simulink model "ECS_FOS"  (Simulink 8.2)
settings: Solver=ode45  StartTime=0.0  StopTime=18000  RelTol=1e-3
InitFcn:
  | load('loss_coeff_mixing_junction.mat')
  | load('SampleOutput.mat')
  | load('HydProp.mat')
  | load('HydraulicLoad.mat')
  | load('initavload.mat')
  | load('SampleFuelBurn.mat')
values from neighbouring files (symbols this model uses):
  FuelBurn = [0 0 0 0 0 0 0 0 0 0 0 0 ... (18249 elements, 1x18249)]    [Benchmark_data1.mat]
  fueltankdata =     [Benchmark_data1.mat]
undefined symbols (not defined in the file or in its folder): AirProp, F1, F2, HUGHES_TREITLER, magnitude, PN_70147, PumpProp
libraries: PowerFlowLib x46, simulink x4
(part 2 of 5)

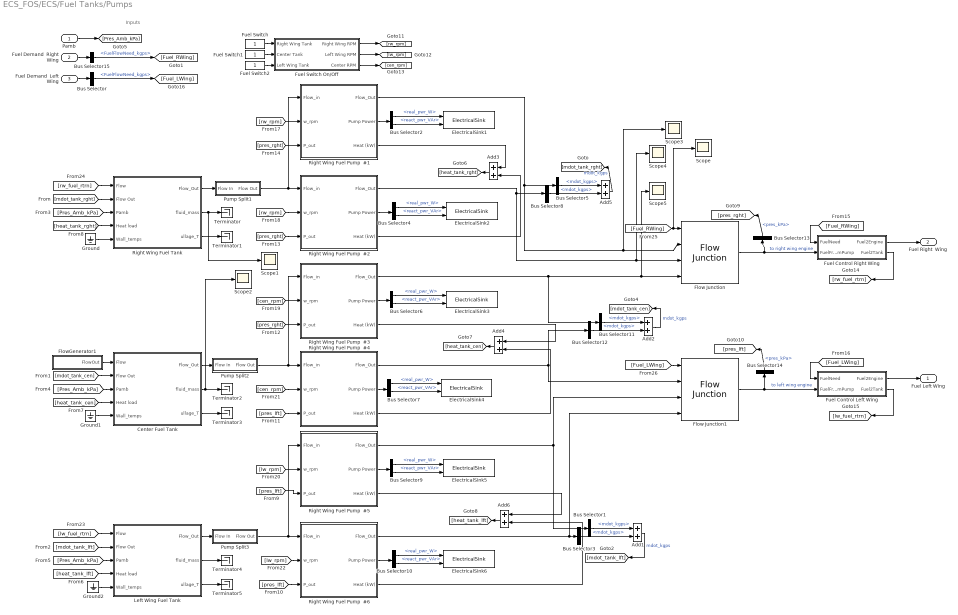
== system ECS_FOS/ECS/Fuel Tanks/Pumps ==
  note: Inputs
  Pamb : Inport
  Fuel Demand  Right Wing : Inport  Port=2
  Fuel Demand  Left Wing : Inport  Port=3
  Add{1..6} (6 alike) : Sum
  Bus Selector : BusSelector  OutputSignals=Fuel.FuelFlowNeed_kgps
  Bus Selector{1,3,5,8,11..12} (6 alike) : BusSelector  OutputSignals=mdot_kgps
  Bus Selector{2,4,6..7,9..10} (6 alike) : BusSelector  OutputSignals=real_pwr_W,react_pwr_VAr
  Bus Selector13 : BusSelector  OutputSignals=pres_kPa
  Bus Selector14 : BusSelector  OutputSignals=pres_kPa
  Bus Selector15 : BusSelector  OutputSignals=Fuel.FuelFlowNeed_kgps
  Center Fuel Tank : Subsystem  AncestorBlock=PowerFlowLib/Energy & Power Systems/Thermal/Fuel/Fuel Tank  mask(Fuel Tank){fileslct=off, filename=fueltank_area.m, filedir=C:\Users\mwillms4\Documents\My Box Files\Graduate\Research\PowerFlow Development\PowerFlow Fall 2013\SupportFunctions\fueltank_area.m, tank_loc=Center Tank, areaprompt2=off, max_vol=3.2, m_init=2500, fld_Tint=0, ull_Tint=30, Pover=100, HTC_fg=14.2, wallHXF=off, wetHTC=14.2, dryHTC=14.2, Qinternal=0}
      mask prompts: fileslct "Browse for area .m file?"; filename "Fuel Tank Area .m File"; filedir "Area .m File Directory"; tank_loc "Select Tank"; areaprompt2 "Edit Fuel Tank Area Manually?"; max_vol "Maximum Tank Volume [m³]"; m_init "Initial Fluid Mass [kg]"; fld_Tint "Initial Fluid Temperature [°C]"; ull_Tint "Initial Ullage Temperature [°C]"; Pover "Tank Pressurization [kPa]"; HTC_fg "Fuel to Ullage HTC [W/m² K]"; wallHXF "Enable Wall Heat Transfer"; wetHTC "Wall to Fluid HTC [W/m² K]"; dryHTC "Wall to Ullage HTC [W/m² K]"; Qinternal "Internal Heat Load [W]"
      mask help:
      | Input 1: Input Flow Bus
      | Input 2: Flow Rate Out [kg/s]
      | Input 3: Ambient Pressure [kPa]
      | Input 4: Heat Load [W]
      | Input 5: Initial Wall Temps. Vector [K]
      |
      | Output 1: Output Flow Bus
      | Output 2: Tank mass [kg]
      | Output 3: Ullage Temp. [K]
      mask init:
      | h      = get_param(gcb,'handle');   % Get block handle
      | blk    = gcb; 
      | hblock = get(h);     % Parse out handles structure 
      | 
      | 
      | %load FluidProperties
      | if exist('F1') == 0
      |     load FluidProp_JetA3638
      |     F1 = FuelProp;
      | end
      | if exist('AirProp') == 0
      |     load AirProp.mat
      | end
      | %{
      | % the following checks for the existance of a file and loads the
      | % spreadsheet into variables that populate the 2D lookup table
      | 
      | if isempty(filedir) == 0;
      |     areadata = xlsread(filedir,1);
      |     vol_per = areadata(:,1);
      |     wall_area = [areadata(:,2:size(areadata,2))];
      | end
      | %}
      | if strcmp(hblock.areaprompt2,'on') == 0;
      |     
      |     % run the selected fuel area file
      |     if ~isempty(strfind(filename,'.m'))
      |         try
      |             run(filename(1:strfind(filename,'.m')-1))       % removing the .m extension and loading the file
      |         catch
      |             error(['Unable to load selected fuel area file in ',blk,'. Verify the file is a .m script file and on the MATLAB Path'])
      |         end
      |     else
      |         try
      |             run(filename)
      |         catch
      |             error(['Unable to load selected fuel area file in ',blk,'. Verify the file is a .m script file and on the MATLAB Path'])
      |         end
      |     end
      |    
      |     switch hblock.tank_loc
      |         case 'Left Wing Tank'
      |             set_param([blk,'/Wall Heat Transfer/volume_%'],'Table', 'fueltankdata.leftwingtank');
      |             %BP1values = strcat('[',num2str(linspace(0,1,size(fueltankdata.leftwingtank,1))),']');
      |             %BP2values = strcat('[',num2str(linspace(1,size(fueltankdata.leftwingtank,2),size(fueltankdata.leftwingtank,2))),']');
      |             set_param([blk,'/Wall Heat Transfer/volume_%'],'BreakpointsForDimension1', 'linspace(0,1,11)');
      |             set_param([blk,'/Wall Heat Transfer/volume_%'],'BreakpointsForDimension2', 'linspace(1,6,6)');
      |             set_param([blk,'/Wall Heat Transfer/Walls 1 to n'],'Value','1:size(fueltankdata.leftwingtank,2)');
      |             set_param([blk,'/Wall Heat Transfer/total area'],'Bias','-[fueltankdata.leftwingtank(11,:)]');
      |             set_param([blk,'/ullage-fluid_area'],'Value','fueltankdata.leftwingtank(2,2)');
      |             
      |         case 'Center Tank'
      |             set_param([blk,'/Wall Heat Transfer/volume_%'],'Table', 'fueltankdata.centertank');
      |             %BP1values = strcat('[',num2str(linspace(0,1,size(fueltankdata.centertank,1))),']');
      |             %BP2values = strcat('[',num2str(linspace(1,size(fueltankdata.centertank,2),size(fueltankdata.centertank,2))),']');
      |             set_param([blk,'/Wall Heat Transfer/volume_%'],'BreakpointsForDimension1', 'linspace(0,1,11)');
      |             set_param([blk,'/Wall Heat Transfer/volume_%'],'BreakpointsForDimension2', 'linspace(1,6,6)');
      |             set_param([blk,'/Wall Heat Transfer/Walls 1 to n'],'Value','1:size(fueltankdata.centertank,2)');
      |             set_param([blk,'/Wall Heat Transfer/total area'],'Bias','-[fueltankdata.centertank(11,:)]');
      |             set_param([blk,'/ullage-fluid_area'],'Value','fueltankdata.centertank(2,2)');
      |             
      |         case 'Right Wing Tank'
      |             set_param([blk,'/Wall Heat Transfer/volume_%'],'Table', 'fueltankdata.rightwingtank');
      |             %BP1values = strcat('[',num2str(linspace(0,1,size(fueltankdata.rightwingtank,1))),']');
      |             %BP2values = strcat('[',num2str(linspace(1,size(fueltankdata.rightwingtank,2),size(fueltankdata.rightwingtank,2))),']');
      |             set_param([blk,'/Wall Heat Transfer/volume_%'],'BreakpointsForDimension1', 'linspace(0,1,11)');
      |             set_param([blk,'/Wall Heat Transfer/volume_%'],'BreakpointsForDimension2', 'linspace(1,6,6)');
      |             set_param([blk,'/Wall Heat Transfer/Walls 1 to n'],'Value','1:size(fueltankdata.rightwingtank,2)');
      |             set_param([blk,'/Wall Heat Transfer/total area'],'Bias','-[fueltankdata.rightwingtank(11,:)]');
      |             set_param([blk,'/ullage-fluid_area'],'Value','fueltankdata.rightwingtank(2,2)');
      |             
      |     end
      |     
      | end
      | 
      | %% CHECK FOR VOLUME OF FUEL BEING GREATER THAN VOLUME OF TANK
      | X = FuelProp.P;
      | Y = FuelProp.T;
      | delx = X(2)-X(1);
      | dely = Y(2)-Y(1);
      | xref = round((Pover + 101 - X(1))/delx);
      | yref = round((fld_Tint + 273 - Y(1))/dely);
      | 
      | rhoIC = FuelProp.Rho_pt(xref,yref);
      | volIC = m_init / rhoIC;
      | 
      | if volIC > max_vol
      |     error('Initial volume of fluid is greater than max volume of tank.')
      | end
      | 
      | 
      | clear h blk hblock
      mask Callback fileslct:
      | h      = get_param(gcb,'handle');   % Get block handle
      | blk    = gcb;
      | hblock = get(h);     % Parse out handles structure
      | 
      | if strcmp(hblock.fileslct,'on') == 1;
      |     set_param(gcb,'areaprompt2','off');     % turn off manual switch
      |     RR_SetPerfSlct(2,0);                    % call uiopen script
      | end
      | 
      | clear h blk hblock
      mask TypeOptions tank_loc: Left Wing Tank | Center Tank | Right Wing Tank
      mask Callback areaprompt2:
      | h      = get_param(gcb,'handle');   % Get block handle
      | blk    = gcb;
      | hblock = get(h);     % Parse out handles structure
      | 
      | if strcmp(hblock.areaprompt2,'on') == 1;
      |     set_param(gcb,'fileslct','off');
      |     open_system([blk, '/Wall Heat Transfer/volume_%']);
      | end
      mask Callback wallHXF:
      | h      = get_param(gcb,'handle');   % Get block handle
      | blk    = gcb;
      | hblock = get(h);     % Parse out handles structure
      | 
      | if strcmp(hblock.wallHXF,'on') == 1;
      |     set_param([blk,'/enable_wall_HXF'],'Value','1');
      | else
      |     set_param([blk,'/enable_wall_HXF'],'Value','0');
      | end
      | 
      | clear h blk hblock
      mask Display:
      | image(imread('fueltank.jpg'))
      | 
      | port_label('input',1,'{\bf Flow In}','TexMode','on')
      | port_label('input',2,'{\bf Flow Rate Out}','TexMode','on')
      | port_label('input',3,'{\bf P_a_m_b [kPa]}','TexMode','on')
      | port_label('input',4,'{\bf Heat Load [kW]}','TexMode','on')
      | port_label('input',5,'{\bf Wall Temp. [K]}','TexMode','on')
      | 
      | port_label('output',1,'{\bf Flow Out }','TexMode','on')
      | port_label('output',2,'{\bf Fluid Mass [kg]}','TexMode','on')
      | port_label('output',3,'{\bf Ullage Temp. [K]}','TexMode','on')
  ElectricalSink1 : PowerFlowLib/Support Functions//Tools/ElectricalSink  Tag=Flow  Description=TwoPhase  load_loc=RightWing  ACDC_load=AC  units=Watts  unq_id=4424
  ElectricalSink2 : PowerFlowLib/Support Functions//Tools/ElectricalSink  Tag=Flow  Description=TwoPhase  load_loc=RightWing  ACDC_load=AC  units=Watts  unq_id=6110
  ElectricalSink3 : PowerFlowLib/Support Functions//Tools/ElectricalSink  Tag=Flow  Description=TwoPhase  load_loc=RightWing  ACDC_load=AC  units=Watts  unq_id=1683
  ElectricalSink4 : PowerFlowLib/Support Functions//Tools/ElectricalSink  Tag=Flow  Description=TwoPhase  load_loc=LeftWing  ACDC_load=AC  units=Watts  unq_id=1485
  ElectricalSink5 : PowerFlowLib/Support Functions//Tools/ElectricalSink  Tag=Flow  Description=TwoPhase  load_loc=LeftWing  ACDC_load=AC  units=Watts  unq_id=5777
  ElectricalSink6 : PowerFlowLib/Support Functions//Tools/ElectricalSink  Tag=Flow  Description=TwoPhase  load_loc=LeftWing  ACDC_load=AC  units=Watts  unq_id=8012
  Flow Junction : PowerFlowLib/Energy & Power Systems/Thermal/Fuel/Flow Junction  Description=TwoPhase  V=.05  Bm=10^5  initPres=6000  initTemp=30
  Flow Junction1 : PowerFlowLib/Energy & Power Systems/Thermal/Fuel/Flow Junction  Description=TwoPhase  V=.05  Bm=10^5  initPres=6000  initTemp=30
  FlowGenerator1 : Subsystem  Tag=Flow  Description=TwoPhase  mask{fld_type1=null, flowrate=0, flowtemp=0, flowpres=00, flowenthalpy=0}
      mask prompts: fld_type1 "Fluid Type"; flowrate "Fluid Flow Rate (kg/s)"; flowtemp "Fluid Flow Temperature (C)"; flowpres "Fluid Flow Pressure (kPa)"; flowenthalpy "Fluid Flow Enthalpy (kJ/kg)"
      mask TypeOptions fld_type1: null
      mask Display: text(.5,.5,'Flow Source','horizontalAlignment','center','texmode','on')
  Fuel Control Left Wing : Subsystem
      mask Display:
      | port_label('input',1,'{\bf Fuel Need}','TexMode','on')
      | port_label('input',2,'{\bf Fuel In}','TexMode','on')
      | 
      | 
      | port_label('output',1,'{\bf Fuel to Eng.}','TexMode','on')
      | port_label('output',2,'{\bf Fuel Return}','TexMode','on')
  "Fuel Control Right Wing " : Subsystem
      mask Display:
      | port_label('input',1,'{\bf Fuel Need}','TexMode','on')
      | port_label('input',2,'{\bf Fuel In}','TexMode','on')
      | 
      | 
      | port_label('output',1,'{\bf Fuel to Eng.}','TexMode','on')
      | port_label('output',2,'{\bf Fuel Return}','TexMode','on')
  Fuel Switch : Constant
  Fuel Switch On/Off : Subsystem
  Fuel Switch1 : Constant
  Fuel Switch2 : Constant
  Ground : Ground
  Ground1 : Ground
  Ground2 : Ground
  Left Wing Fuel Tank : Subsystem  AncestorBlock=PowerFlowLib/Energy & Power Systems/Thermal/Fuel/Fuel Tank  mask(Fuel Tank){fileslct=off, filename=fueltank_area.m, filedir=C:\Users\mwillms4\Documents\My Box Files\Graduate\Research\PowerFlow Development\PowerFlow Fall 2013\SupportFunctions\fueltank_area.m, tank_loc=Left Wing Tank, areaprompt2=off, max_vol=3.2, m_init=2500, fld_Tint=0, ull_Tint=30, Pover=100, HTC_fg=14.2, wallHXF=off, wetHTC=14.2, dryHTC=14.2, Qinternal=0}
      mask prompts: fileslct "Browse for area .m file?"; filename "Fuel Tank Area .m File"; filedir "Area .m File Directory"; tank_loc "Select Tank"; areaprompt2 "Edit Fuel Tank Area Manually?"; max_vol "Maximum Tank Volume [m³]"; m_init "Initial Fluid Mass [kg]"; fld_Tint "Initial Fluid Temperature [°C]"; ull_Tint "Initial Ullage Temperature [°C]"; Pover "Tank Pressurization [kPa]"; HTC_fg "Fuel to Ullage HTC [W/m² K]"; wallHXF "Enable Wall Heat Transfer"; wetHTC "Wall to Fluid HTC [W/m² K]"; dryHTC "Wall to Ullage HTC [W/m² K]"; Qinternal "Internal Heat Load [W]"
      mask help:
      | Input 1: Input Flow Bus
      | Input 2: Flow Rate Out [kg/s]
      | Input 3: Ambient Pressure [kPa]
      | Input 4: Heat Load [W]
      | Input 5: Initial Wall Temps. Vector [K]
      |
      | Output 1: Output Flow Bus
      | Output 2: Tank mass [kg]
      | Output 3: Ullage Temp. [K]
      mask init: same as ECS_FOS/ECS/Fuel Tanks/Pumps/Center Fuel Tank
      mask Callback fileslct:
      | h      = get_param(gcb,'handle');   % Get block handle
      | blk    = gcb;
      | hblock = get(h);     % Parse out handles structure
      | 
      | if strcmp(hblock.fileslct,'on') == 1;
      |     set_param(gcb,'areaprompt2','off');     % turn off manual switch
      |     RR_SetPerfSlct(2,0);                    % call uiopen script
      | end
      | 
      | clear h blk hblock
      mask TypeOptions tank_loc: Left Wing Tank | Center Tank | Right Wing Tank
      mask Callback areaprompt2:
      | h      = get_param(gcb,'handle');   % Get block handle
      | blk    = gcb;
      | hblock = get(h);     % Parse out handles structure
      | 
      | if strcmp(hblock.areaprompt2,'on') == 1;
      |     set_param(gcb,'fileslct','off');
      |     open_system([blk, '/Wall Heat Transfer/volume_%']);
      | end
      mask Callback wallHXF:
      | h      = get_param(gcb,'handle');   % Get block handle
      | blk    = gcb;
      | hblock = get(h);     % Parse out handles structure
      | 
      | if strcmp(hblock.wallHXF,'on') == 1;
      |     set_param([blk,'/enable_wall_HXF'],'Value','1');
      | else
      |     set_param([blk,'/enable_wall_HXF'],'Value','0');
      | end
      | 
      | clear h blk hblock
      mask Display:
      | image(imread('fueltank.jpg'))
      | 
      | port_label('input',1,'{\bf Flow In}','TexMode','on')
      | port_label('input',2,'{\bf Flow Rate Out}','TexMode','on')
      | port_label('input',3,'{\bf P_a_m_b [kPa]}','TexMode','on')
      | port_label('input',4,'{\bf Heat Load [kW]}','TexMode','on')
      | port_label('input',5,'{\bf Wall Temp. [K]}','TexMode','on')
      | 
      | port_label('output',1,'{\bf Flow Out }','TexMode','on')
      | port_label('output',2,'{\bf Fluid Mass [kg]}','TexMode','on')
      | port_label('output',3,'{\bf Ullage Temp. [K]}','TexMode','on')
  Pump Split1 : Subsystem
  Pump Split2 : Subsystem
  Pump Split3 : Subsystem
  Right Wing Fuel Pump  #1 : Subsystem  AncestorBlock=PowerFlowLib/Energy & Power Systems/Thermal/Fuel/Fuel Pump  mask(Pump){maptype=Pressure (kPa) vs. Vol. Flow Rate (m³/hr), map=B737_AC_fuel1, map_load=off, SG=0.82, pump_eff=.75, heat_out=off, AC_pwr=on, pf=1, mech_pwr=off}
      mask prompts: maptype "Map Type"; map "Select Map"; map_load "Load new map?"; SG "Specific Gravity of Flow"; pump_eff "Pump Overall Efficiency"; heat_out "Add heat to flow?"; AC_pwr "AC Powered?"; pf "Power Factor"; mech_pwr "Mechanically Driven?"
      mask help:
      | Input 1: Input Flow Bus
      | Input 2: Shaft RPM (rpm)
      | Input 3: Upstream Pressure (kPa)
      |
      | Output 1: Output Flow Bus
      | Output 2: Pump Power Bus (mech or elec)
      | Optional: Pump Heat Generated (kW)
      mask init:
      | h      = get_param(gcb,'handle');   % Get block handle
      | blk    = gcb; 
      | hblock = get(h);     % Parse out handles structure 
      | 
      | if exist('PumpProp') == 0
      |   load('PumpProp.mat')
      | end
      | 
      | if strcmp(hblock.maptype,'Head (m) vs. Vol. Flow Rate (m³/hr)') == 1;
      |     set_param([blk,'/switchcase'],'Value','1');
      |     set_param([blk,'/Pump Vol. FlowRate'],'Table',['PumpProp.',map,'.q']);
      |     set_param([blk,'/Pump Vol. FlowRate'],'BreakpointsForDimension1',['PumpProp.',map,'.head']);
      | elseif strcmp(hblock.maptype,'Pressure (kPa) vs. Vol. Flow Rate (m³/hr)') == 1;
      |     set_param([blk,'/switchcase'],'Value','2');
      |     set_param([blk,'/Pump Vol. FlowRate'],'Table',['PumpProp.',map,'.q']);
      |     set_param([blk,'/Pump Vol. FlowRate'],'BreakpointsForDimension1',['PumpProp.',map,'.pres']);
      | elseif strcmp(hblock.maptype,'Pressure (bar) vs. Vol. Flow Rate (m³/hr)') == 1;
      |     set_param([blk,'/switchcase'],'Value','3');
      |     set_param([blk,'/Pump Vol. FlowRate'],'Table',['PumpProp.',map,'.q']);
      |     set_param([blk,'/Pump Vol. FlowRate'],'BreakpointsForDimension1',['PumpProp.',map,'.pres']);
      | else
      |     error('see pump mask callback for map type');
      | end    
      | 
      | % TURNING ON/OFF PUMP HEAT GENERATION OUTPUT
      | if strcmp(hblock.heat_out,'on') == 1;   % adding heat to fluid flow
      |     set_param([blk,'/heat_switch'],'Gain','1')  % turn on heat added to flow
      |     try
      |         delete_block([blk,'/Heat (kW)'])
      |     catch
      |     end
      |     delete_unconnected_lines(blk)
      |         
      | elseif strcmp(hblock.heat_out,'off') == 1; % not adding heat to fluid flow
      |     set_param([blk,'/heat_switch'],'Gain','0')  % adding no heat to flow
      |     try
      |         add_block('built-in/Outport',[blk,'/Heat (kW)'],'Position',[800 200 830 214]);
      |         add_line(blk,'W to kW/1','Heat (kW)/1')
      |     catch
      |     end
      | end
      | 
      | clear h blk hblock
      settings: OpenFcn=|
      | if exist('PumpProp') == 0
      |   load('PumpProp.mat')
      | end
      | open_system(gcb,'mask')
      mask TypeOptions maptype: Head (m) vs. Vol. Flow Rate (m³/hr) | Pressure (kPa) vs. Vol. Flow Rate (m³/hr) | Pressure (bar) vs. Vol. Flow Rate (m³/hr)
      mask Callback maptype:
      | h      = get_param(gcb,'handle');   % Get block handle
      | blk    = gcb;
      | hblock = get(h);     % Parse out handles structure
      | 
      | if strcmp(hblock.maptype,'Head (m) vs. Vol. Flow Rate (m³/hr)') == 1;
      |     set_param([blk,'/switchcase'],'Value','1');
      |     set_param([blk,'/Pump Vol. FlowRate'],'Table',['PumpProp.',hblock.map,'.q']);
      |     set_param([blk,'/Pump Vol. FlowRate'],'BreakpointsForDimension1',['PumpProp.',hblock.map,'.head']);
      | elseif strcmp(hblock.maptype,'Pressure (kPa) vs. Vol. Flow Rate (m³/hr)') == 1;
      |     set_param([blk,'/switchcase'],'Value','2');
      |     set_param([blk,'/Pump Vol. FlowRate'],'Table',['PumpProp.',hblock.map,'.q']);
      |     set_param([blk,'/Pump Vol. FlowRate'],'BreakpointsForDimension1',['PumpProp.',hblock.map,'.pres']);
      | elseif strcmp(hblock.maptype,'Pressure (bar) vs. Vol. Flow Rate (m³/hr)') == 1;
      |     set_param([blk,'/switchcase'],'Value','3');
      |     set_param([blk,'/Pump Vol. FlowRate'],'Table',['PumpProp.',hblock.map,'.q']);
      |     set_param([blk,'/Pump Vol. FlowRate'],'BreakpointsForDimension1',['PumpProp.',hblock.map,'.pres']);
      | else
      |     error('see pump mask callback for map type');
      | end
      | 
      | clear h blk hblock
      mask TypeOptions map: B737_mech_fuel1 | B737_mech_fuel2 | B737_mech_fuel3 | B737_AC_fuel1 | B737_AC_oil1
      mask Callback map:
      | h      = get_param(gcb,'handle');   % Get block handle
      | blk    = gcb;
      | hblock = get(h);     % Parse out handles structure
      | vals = get_param(blk,'MaskValues');
      | % find all installed pumps in the PumpProp.mat file
      | pumps = fieldnames(PumpProp);
      | indx = strfind(pumps, 'units');
      | indx = find(not(cellfun('isempty', indx)));
      | pumps(indx) = [];      % removing the units entry
      | 
      | for i = 1:size(pumps,1);
      |    if i==1;
      |     pmpstr = pumps{i};
      |    else
      |        pmpstr = strcat(pmpstr,char(124),pumps{i});
      |    end
      | end
      | 
      | % Get the mask parameter values. This is a cell array of strings.
      | styl = get_param(blk,'MaskStyles');
      | 
      | vis = get_param(blk,'MaskVisibilities');
      | str = get_param(blk,'MaskPromptString');
      | 
      | % fill the mask with the parameters
      | set_param(blk,'MaskVisibilities',vis,'MaskPromptString',str,'MaskValues',vals,'MaskStyles',[styl(1);strcat('popup(',pmpstr,')');styl(3:9)]);
      | 
      | clear h blk hblock styl vals vis str pmpstr i indx pumps
      mask Callback AC_pwr:
      | h      = get_param(gcb,'handle');   % Get block handle
      | blk    = gcb;
      | hblock = get(h);     % Parse out handles structure
      | 
      | vis = get_param(blk,'MaskVisibilities');
      | 
      | if strcmp(hblock.AC_pwr,'off') == 1;
      |     % fill the mask with the parameters
      |     set_param(blk,'MaskVisibilities',[vis(1:7);'off';vis(9)])
      |     set_param(blk,'mech_pwr','on');
      |     set_param([blk,'/pwr_switch'],'Value','0.5')
      | elseif strcmp(hblock.AC_pwr,'on') == 1;
      |     % fill the mask with the parameters
      |     set_param(blk,'MaskVisibilities',[vis(1:7);'on';vis(9)])
      |     set_param(blk,'mech_pwr','off');
      |     set_param([blk,'/pwr_switch'],'Value','0')
      | end
      | 
      | clear h blk hblock vis
      mask Callback mech_pwr:
      | h      = get_param(gcb,'handle');   % Get block handle
      | blk    = gcb;
      | hblock = get(h);     % Parse out handles structure
      | 
      | vis = get_param(blk,'MaskVisibilities');
      | 
      | if strcmp(hblock.mech_pwr,'off') == 1;
      |     % fill the mask with the parameters
      |     set_param(blk,'MaskVisibilities',[vis(1:7);'on';vis(9)])
      |     set_param(blk,'AC_pwr','on');
      |     set_param([blk,'/pwr_switch'],'Value','0')
      | elseif strcmp(hblock.mech_pwr,'on') == 1;
      |     % fill the mask with the parameters
      |     set_param(blk,'MaskVisibilities',[vis(1:7);'off';vis(9)])
      |     set_param(blk,'AC_pwr','off');
      |     set_param([blk,'/pwr_switch'],'Value','0.5')
      | end
      | clear h blk hblock vis
      mask Display:
      | image(imread('centpump.jpg'));
      | 
      | port_label('input',1,'{\bf Flow In}','TexMode','on')
      | port_label('input',2,'{\bf w (rpm)}','TexMode','on')
      | port_label('input',3,'{\bf P_o_u_t (kPa)}','TexMode','on')
      | 
      | port_label('output',1,'{\bf Flow Out}','TexMode','on')
      | port_label('output',2,'{\bf Pump Power}','TexMode','on')
      | 
      | h      = get_param(gcb,'handle');   % Get block handle
      | hblock = get(h);     % Parse out handles structure
      | 
      | if heat_out == 0
      |     port_label('output',3,'{\bf Pump Heat [kW]}','TexMode','on')
      | end
  Right Wing Fuel Pump  #2 : Subsystem  AncestorBlock=PowerFlowLib/Energy & Power Systems/Thermal/Fuel/Fuel Pump  mask(Pump){maptype=Pressure (kPa) vs. Vol. Flow Rate (m³/hr), map=B737_AC_fuel1, map_load=off, SG=0.82, pump_eff=.75, heat_out=off, AC_pwr=on, pf=1, mech_pwr=off}
      mask prompts: maptype "Map Type"; map "Select Map"; map_load "Load new map?"; SG "Specific Gravity of Flow"; pump_eff "Pump Overall Efficiency"; heat_out "Add heat to flow?"; AC_pwr "AC Powered?"; pf "Power Factor"; mech_pwr "Mechanically Driven?"
      mask help:
      | Input 1: Input Flow Bus
      | Input 2: Shaft RPM (rpm)
      | Input 3: Upstream Pressure (kPa)
      |
      | Output 1: Output Flow Bus
      | Output 2: Pump Power Bus (mech or elec)
      | Optional: Pump Heat Generated (kW)
      mask init: same as ECS_FOS/ECS/Fuel Tanks/Pumps/Right Wing Fuel Pump  #1
      settings: OpenFcn=|
      | if exist('PumpProp') == 0
      |   load('PumpProp.mat')
      | end
      | open_system(gcb,'mask')
      mask TypeOptions maptype: Head (m) vs. Vol. Flow Rate (m³/hr) | Pressure (kPa) vs. Vol. Flow Rate (m³/hr) | Pressure (bar) vs. Vol. Flow Rate (m³/hr)
      mask Callback maptype:
      | h      = get_param(gcb,'handle');   % Get block handle
      | blk    = gcb;
      | hblock = get(h);     % Parse out handles structure
      | 
      | if strcmp(hblock.maptype,'Head (m) vs. Vol. Flow Rate (m³/hr)') == 1;
      |     set_param([blk,'/switchcase'],'Value','1');
      |     set_param([blk,'/Pump Vol. FlowRate'],'Table',['PumpProp.',hblock.map,'.q']);
      |     set_param([blk,'/Pump Vol. FlowRate'],'BreakpointsForDimension1',['PumpProp.',hblock.map,'.head']);
      | elseif strcmp(hblock.maptype,'Pressure (kPa) vs. Vol. Flow Rate (m³/hr)') == 1;
      |     set_param([blk,'/switchcase'],'Value','2');
      |     set_param([blk,'/Pump Vol. FlowRate'],'Table',['PumpProp.',hblock.map,'.q']);
      |     set_param([blk,'/Pump Vol. FlowRate'],'BreakpointsForDimension1',['PumpProp.',hblock.map,'.pres']);
      | elseif strcmp(hblock.maptype,'Pressure (bar) vs. Vol. Flow Rate (m³/hr)') == 1;
      |     set_param([blk,'/switchcase'],'Value','3');
      |     set_param([blk,'/Pump Vol. FlowRate'],'Table',['PumpProp.',hblock.map,'.q']);
      |     set_param([blk,'/Pump Vol. FlowRate'],'BreakpointsForDimension1',['PumpProp.',hblock.map,'.pres']);
      | else
      |     error('see pump mask callback for map type');
      | end
      | 
      | clear h blk hblock
      mask TypeOptions map: B737_mech_fuel1 | B737_mech_fuel2 | B737_mech_fuel3 | B737_AC_fuel1 | B737_AC_oil1
      mask Callback map:
      | h      = get_param(gcb,'handle');   % Get block handle
      | blk    = gcb;
      | hblock = get(h);     % Parse out handles structure
      | vals = get_param(blk,'MaskValues');
      | % find all installed pumps in the PumpProp.mat file
      | pumps = fieldnames(PumpProp);
      | indx = strfind(pumps, 'units');
      | indx = find(not(cellfun('isempty', indx)));
      | pumps(indx) = [];      % removing the units entry
      | 
      | for i = 1:size(pumps,1);
      |    if i==1;
      |     pmpstr = pumps{i};
      |    else
      |        pmpstr = strcat(pmpstr,char(124),pumps{i});
      |    end
      | end
      | 
      | % Get the mask parameter values. This is a cell array of strings.
      | styl = get_param(blk,'MaskStyles');
      | 
      | vis = get_param(blk,'MaskVisibilities');
      | str = get_param(blk,'MaskPromptString');
      | 
      | % fill the mask with the parameters
      | set_param(blk,'MaskVisibilities',vis,'MaskPromptString',str,'MaskValues',vals,'MaskStyles',[styl(1);strcat('popup(',pmpstr,')');styl(3:9)]);
      | 
      | clear h blk hblock styl vals vis str pmpstr i indx pumps
      mask Callback AC_pwr:
      | h      = get_param(gcb,'handle');   % Get block handle
      | blk    = gcb;
      | hblock = get(h);     % Parse out handles structure
      | 
      | vis = get_param(blk,'MaskVisibilities');
      | 
      | if strcmp(hblock.AC_pwr,'off') == 1;
      |     % fill the mask with the parameters
      |     set_param(blk,'MaskVisibilities',[vis(1:7);'off';vis(9)])
      |     set_param(blk,'mech_pwr','on');
      |     set_param([blk,'/pwr_switch'],'Value','0.5')
      | elseif strcmp(hblock.AC_pwr,'on') == 1;
      |     % fill the mask with the parameters
      |     set_param(blk,'MaskVisibilities',[vis(1:7);'on';vis(9)])
      |     set_param(blk,'mech_pwr','off');
      |     set_param([blk,'/pwr_switch'],'Value','0')
      | end
      | 
      | clear h blk hblock vis
      mask Callback mech_pwr:
      | h      = get_param(gcb,'handle');   % Get block handle
      | blk    = gcb;
      | hblock = get(h);     % Parse out handles structure
      | 
      | vis = get_param(blk,'MaskVisibilities');
      | 
      | if strcmp(hblock.mech_pwr,'off') == 1;
      |     % fill the mask with the parameters
      |     set_param(blk,'MaskVisibilities',[vis(1:7);'on';vis(9)])
      |     set_param(blk,'AC_pwr','on');
      |     set_param([blk,'/pwr_switch'],'Value','0')
      | elseif strcmp(hblock.mech_pwr,'on') == 1;
      |     % fill the mask with the parameters
      |     set_param(blk,'MaskVisibilities',[vis(1:7);'off';vis(9)])
      |     set_param(blk,'AC_pwr','off');
      |     set_param([blk,'/pwr_switch'],'Value','0.5')
      | end
      | clear h blk hblock vis
      mask Display:
      | image(imread('centpump.jpg'));
      | 
      | port_label('input',1,'{\bf Flow In}','TexMode','on')
      | port_label('input',2,'{\bf w (rpm)}','TexMode','on')
      | port_label('input',3,'{\bf P_o_u_t (kPa)}','TexMode','on')
      | 
      | port_label('output',1,'{\bf Flow Out}','TexMode','on')
      | port_label('output',2,'{\bf Pump Power}','TexMode','on')
      | 
      | h      = get_param(gcb,'handle');   % Get block handle
      | hblock = get(h);     % Parse out handles structure
      | 
      | if heat_out == 0
      |     port_label('output',3,'{\bf Pump Heat [kW]}','TexMode','on')
      | end
  Right Wing Fuel Pump  #3 : Subsystem  AncestorBlock=PowerFlowLib/Energy & Power Systems/Thermal/Fuel/Fuel Pump  mask(Pump){maptype=Pressure (kPa) vs. Vol. Flow Rate (m³/hr), map=B737_AC_fuel1, map_load=off, SG=0.82, pump_eff=.75, heat_out=off, AC_pwr=on, pf=1, mech_pwr=off}
      mask prompts: maptype "Map Type"; map "Select Map"; map_load "Load new map?"; SG "Specific Gravity of Flow"; pump_eff "Pump Overall Efficiency"; heat_out "Add heat to flow?"; AC_pwr "AC Powered?"; pf "Power Factor"; mech_pwr "Mechanically Driven?"
      mask help:
      | Input 1: Input Flow Bus
      | Input 2: Shaft RPM (rpm)
      | Input 3: Upstream Pressure (kPa)
      |
      | Output 1: Output Flow Bus
      | Output 2: Pump Power Bus (mech or elec)
      | Optional: Pump Heat Generated (kW)
      mask init: same as ECS_FOS/ECS/Fuel Tanks/Pumps/Right Wing Fuel Pump  #1
      settings: OpenFcn=|
      | if exist('PumpProp') == 0
      |   load('PumpProp.mat')
      | end
      | open_system(gcb,'mask')
      mask TypeOptions maptype: Head (m) vs. Vol. Flow Rate (m³/hr) | Pressure (kPa) vs. Vol. Flow Rate (m³/hr) | Pressure (bar) vs. Vol. Flow Rate (m³/hr)
      mask Callback maptype:
      | h      = get_param(gcb,'handle');   % Get block handle
      | blk    = gcb;
      | hblock = get(h);     % Parse out handles structure
      | 
      | if strcmp(hblock.maptype,'Head (m) vs. Vol. Flow Rate (m³/hr)') == 1;
      |     set_param([blk,'/switchcase'],'Value','1');
      |     set_param([blk,'/Pump Vol. FlowRate'],'Table',['PumpProp.',hblock.map,'.q']);
      |     set_param([blk,'/Pump Vol. FlowRate'],'BreakpointsForDimension1',['PumpProp.',hblock.map,'.head']);
      | elseif strcmp(hblock.maptype,'Pressure (kPa) vs. Vol. Flow Rate (m³/hr)') == 1;
      |     set_param([blk,'/switchcase'],'Value','2');
      |     set_param([blk,'/Pump Vol. FlowRate'],'Table',['PumpProp.',hblock.map,'.q']);
      |     set_param([blk,'/Pump Vol. FlowRate'],'BreakpointsForDimension1',['PumpProp.',hblock.map,'.pres']);
      | elseif strcmp(hblock.maptype,'Pressure (bar) vs. Vol. Flow Rate (m³/hr)') == 1;
      |     set_param([blk,'/switchcase'],'Value','3');
      |     set_param([blk,'/Pump Vol. FlowRate'],'Table',['PumpProp.',hblock.map,'.q']);
      |     set_param([blk,'/Pump Vol. FlowRate'],'BreakpointsForDimension1',['PumpProp.',hblock.map,'.pres']);
      | else
      |     error('see pump mask callback for map type');
      | end
      | 
      | clear h blk hblock
      mask TypeOptions map: B737_mech_fuel1 | B737_mech_fuel2 | B737_mech_fuel3 | B737_AC_fuel1 | B737_AC_oil1
      mask Callback map:
      | h      = get_param(gcb,'handle');   % Get block handle
      | blk    = gcb;
      | hblock = get(h);     % Parse out handles structure
      | vals = get_param(blk,'MaskValues');
      | % find all installed pumps in the PumpProp.mat file
      | pumps = fieldnames(PumpProp);
      | indx = strfind(pumps, 'units');
      | indx = find(not(cellfun('isempty', indx)));
      | pumps(indx) = [];      % removing the units entry
      | 
      | for i = 1:size(pumps,1);
      |    if i==1;
      |     pmpstr = pumps{i};
      |    else
      |        pmpstr = strcat(pmpstr,char(124),pumps{i});
      |    end
      | end
      | 
      | % Get the mask parameter values. This is a cell array of strings.
      | styl = get_param(blk,'MaskStyles');
      | 
      | vis = get_param(blk,'MaskVisibilities');
      | str = get_param(blk,'MaskPromptString');
      | 
      | % fill the mask with the parameters
      | set_param(blk,'MaskVisibilities',vis,'MaskPromptString',str,'MaskValues',vals,'MaskStyles',[styl(1);strcat('popup(',pmpstr,')');styl(3:9)]);
      | 
      | clear h blk hblock styl vals vis str pmpstr i indx pumps
      mask Callback AC_pwr:
      | h      = get_param(gcb,'handle');   % Get block handle
      | blk    = gcb;
      | hblock = get(h);     % Parse out handles structure
      | 
      | vis = get_param(blk,'MaskVisibilities');
      | 
      | if strcmp(hblock.AC_pwr,'off') == 1;
      |     % fill the mask with the parameters
      |     set_param(blk,'MaskVisibilities',[vis(1:7);'off';vis(9)])
      |     set_param(blk,'mech_pwr','on');
      |     set_param([blk,'/pwr_switch'],'Value','0.5')
      | elseif strcmp(hblock.AC_pwr,'on') == 1;
      |     % fill the mask with the parameters
      |     set_param(blk,'MaskVisibilities',[vis(1:7);'on';vis(9)])
      |     set_param(blk,'mech_pwr','off');
      |     set_param([blk,'/pwr_switch'],'Value','0')
      | end
      | 
      | clear h blk hblock vis
      mask Callback mech_pwr:
      | h      = get_param(gcb,'handle');   % Get block handle
      | blk    = gcb;
      | hblock = get(h);     % Parse out handles structure
      | 
      | vis = get_param(blk,'MaskVisibilities');
      | 
      | if strcmp(hblock.mech_pwr,'off') == 1;
      |     % fill the mask with the parameters
      |     set_param(blk,'MaskVisibilities',[vis(1:7);'on';vis(9)])
      |     set_param(blk,'AC_pwr','on');
      |     set_param([blk,'/pwr_switch'],'Value','0')
      | elseif strcmp(hblock.mech_pwr,'on') == 1;
      |     % fill the mask with the parameters
      |     set_param(blk,'MaskVisibilities',[vis(1:7);'off';vis(9)])
      |     set_param(blk,'AC_pwr','off');
      |     set_param([blk,'/pwr_switch'],'Value','0.5')
      | end
      | clear h blk hblock vis
      mask Display:
      | image(imread('centpump.jpg'));
      | 
      | port_label('input',1,'{\bf Flow In}','TexMode','on')
      | port_label('input',2,'{\bf w (rpm)}','TexMode','on')
      | port_label('input',3,'{\bf P_o_u_t (kPa)}','TexMode','on')
      | 
      | port_label('output',1,'{\bf Flow Out}','TexMode','on')
      | port_label('output',2,'{\bf Pump Power}','TexMode','on')
      | 
      | h      = get_param(gcb,'handle');   % Get block handle
      | hblock = get(h);     % Parse out handles structure
      | 
      | if heat_out == 0
      |     port_label('output',3,'{\bf Pump Heat [kW]}','TexMode','on')
      | end
  Right Wing Fuel Pump  #4 : Subsystem  AncestorBlock=PowerFlowLib/Energy & Power Systems/Thermal/Fuel/Fuel Pump  mask(Pump){maptype=Pressure (kPa) vs. Vol. Flow Rate (m³/hr), map=B737_AC_fuel1, map_load=off, SG=0.82, pump_eff=.75, heat_out=off, AC_pwr=on, pf=1, mech_pwr=off}
      mask prompts: maptype "Map Type"; map "Select Map"; map_load "Load new map?"; SG "Specific Gravity of Flow"; pump_eff "Pump Overall Efficiency"; heat_out "Add heat to flow?"; AC_pwr "AC Powered?"; pf "Power Factor"; mech_pwr "Mechanically Driven?"
      mask help:
      | Input 1: Input Flow Bus
      | Input 2: Shaft RPM (rpm)
      | Input 3: Upstream Pressure (kPa)
      |
      | Output 1: Output Flow Bus
      | Output 2: Pump Power Bus (mech or elec)
      | Optional: Pump Heat Generated (kW)
      mask init: same as ECS_FOS/ECS/Fuel Tanks/Pumps/Right Wing Fuel Pump  #1
      settings: OpenFcn=|
      | if exist('PumpProp') == 0
      |   load('PumpProp.mat')
      | end
      | open_system(gcb,'mask')
      mask TypeOptions maptype: Head (m) vs. Vol. Flow Rate (m³/hr) | Pressure (kPa) vs. Vol. Flow Rate (m³/hr) | Pressure (bar) vs. Vol. Flow Rate (m³/hr)
      mask Callback maptype:
      | h      = get_param(gcb,'handle');   % Get block handle
      | blk    = gcb;
      | hblock = get(h);     % Parse out handles structure
      | 
      | if strcmp(hblock.maptype,'Head (m) vs. Vol. Flow Rate (m³/hr)') == 1;
      |     set_param([blk,'/switchcase'],'Value','1');
      |     set_param([blk,'/Pump Vol. FlowRate'],'Table',['PumpProp.',hblock.map,'.q']);
      |     set_param([blk,'/Pump Vol. FlowRate'],'BreakpointsForDimension1',['PumpProp.',hblock.map,'.head']);
      | elseif strcmp(hblock.maptype,'Pressure (kPa) vs. Vol. Flow Rate (m³/hr)') == 1;
      |     set_param([blk,'/switchcase'],'Value','2');
      |     set_param([blk,'/Pump Vol. FlowRate'],'Table',['PumpProp.',hblock.map,'.q']);
      |     set_param([blk,'/Pump Vol. FlowRate'],'BreakpointsForDimension1',['PumpProp.',hblock.map,'.pres']);
      | elseif strcmp(hblock.maptype,'Pressure (bar) vs. Vol. Flow Rate (m³/hr)') == 1;
      |     set_param([blk,'/switchcase'],'Value','3');
      |     set_param([blk,'/Pump Vol. FlowRate'],'Table',['PumpProp.',hblock.map,'.q']);
      |     set_param([blk,'/Pump Vol. FlowRate'],'BreakpointsForDimension1',['PumpProp.',hblock.map,'.pres']);
      | else
      |     error('see pump mask callback for map type');
      | end
      | 
      | clear h blk hblock
      mask TypeOptions map: B737_mech_fuel1 | B737_mech_fuel2 | B737_mech_fuel3 | B737_AC_fuel1 | B737_AC_oil1
      mask Callback map:
      | h      = get_param(gcb,'handle');   % Get block handle
      | blk    = gcb;
      | hblock = get(h);     % Parse out handles structure
      | vals = get_param(blk,'MaskValues');
      | % find all installed pumps in the PumpProp.mat file
      | pumps = fieldnames(PumpProp);
      | indx = strfind(pumps, 'units');
      | indx = find(not(cellfun('isempty', indx)));
      | pumps(indx) = [];      % removing the units entry
      | 
      | for i = 1:size(pumps,1);
      |    if i==1;
      |     pmpstr = pumps{i};
      |    else
      |        pmpstr = strcat(pmpstr,char(124),pumps{i});
      |    end
      | end
      | 
      | % Get the mask parameter values. This is a cell array of strings.
      | styl = get_param(blk,'MaskStyles');
      | 
      | vis = get_param(blk,'MaskVisibilities');
      | str = get_param(blk,'MaskPromptString');
      | 
      | % fill the mask with the parameters
      | set_param(blk,'MaskVisibilities',vis,'MaskPromptString',str,'MaskValues',vals,'MaskStyles',[styl(1);strcat('popup(',pmpstr,')');styl(3:9)]);
      | 
      | clear h blk hblock styl vals vis str pmpstr i indx pumps
      mask Callback AC_pwr:
      | h      = get_param(gcb,'handle');   % Get block handle
      | blk    = gcb;
      | hblock = get(h);     % Parse out handles structure
      | 
      | vis = get_param(blk,'MaskVisibilities');
      | 
      | if strcmp(hblock.AC_pwr,'off') == 1;
      |     % fill the mask with the parameters
      |     set_param(blk,'MaskVisibilities',[vis(1:7);'off';vis(9)])
      |     set_param(blk,'mech_pwr','on');
      |     set_param([blk,'/pwr_switch'],'Value','0.5')
      | elseif strcmp(hblock.AC_pwr,'on') == 1;
      |     % fill the mask with the parameters
      |     set_param(blk,'MaskVisibilities',[vis(1:7);'on';vis(9)])
      |     set_param(blk,'mech_pwr','off');
      |     set_param([blk,'/pwr_switch'],'Value','0')
      | end
      | 
      | clear h blk hblock vis
      mask Callback mech_pwr:
      | h      = get_param(gcb,'handle');   % Get block handle
      | blk    = gcb;
      | hblock = get(h);     % Parse out handles structure
      | 
      | vis = get_param(blk,'MaskVisibilities');
      | 
      | if strcmp(hblock.mech_pwr,'off') == 1;
      |     % fill the mask with the parameters
      |     set_param(blk,'MaskVisibilities',[vis(1:7);'on';vis(9)])
      |     set_param(blk,'AC_pwr','on');
      |     set_param([blk,'/pwr_switch'],'Value','0')
      | elseif strcmp(hblock.mech_pwr,'on') == 1;
      |     % fill the mask with the parameters
      |     set_param(blk,'MaskVisibilities',[vis(1:7);'off';vis(9)])
      |     set_param(blk,'AC_pwr','off');
      |     set_param([blk,'/pwr_switch'],'Value','0.5')
      | end
      | clear h blk hblock vis
      mask Display:
      | image(imread('centpump.jpg'));
      | 
      | port_label('input',1,'{\bf Flow In}','TexMode','on')
      | port_label('input',2,'{\bf w (rpm)}','TexMode','on')
      | port_label('input',3,'{\bf P_o_u_t (kPa)}','TexMode','on')
      | 
      | port_label('output',1,'{\bf Flow Out}','TexMode','on')
      | port_label('output',2,'{\bf Pump Power}','TexMode','on')
      | 
      | h      = get_param(gcb,'handle');   % Get block handle
      | hblock = get(h);     % Parse out handles structure
      | 
      | if heat_out == 0
      |     port_label('output',3,'{\bf Pump Heat [kW]}','TexMode','on')
      | end
  Right Wing Fuel Pump  #5 : Subsystem  AncestorBlock=PowerFlowLib/Energy & Power Systems/Thermal/Fuel/Fuel Pump  mask(Pump){maptype=Pressure (kPa) vs. Vol. Flow Rate (m³/hr), map=B737_AC_fuel1, map_load=off, SG=0.82, pump_eff=.75, heat_out=off, AC_pwr=on, pf=1, mech_pwr=off}
      mask prompts: maptype "Map Type"; map "Select Map"; map_load "Load new map?"; SG "Specific Gravity of Flow"; pump_eff "Pump Overall Efficiency"; heat_out "Add heat to flow?"; AC_pwr "AC Powered?"; pf "Power Factor"; mech_pwr "Mechanically Driven?"
      mask help:
      | Input 1: Input Flow Bus
      | Input 2: Shaft RPM (rpm)
      | Input 3: Upstream Pressure (kPa)
      |
      | Output 1: Output Flow Bus
      | Output 2: Pump Power Bus (mech or elec)
      | Optional: Pump Heat Generated (kW)
      mask init: same as ECS_FOS/ECS/Fuel Tanks/Pumps/Right Wing Fuel Pump  #1
      settings: OpenFcn=|
      | if exist('PumpProp') == 0
      |   load('PumpProp.mat')
      | end
      | open_system(gcb,'mask')
      mask TypeOptions maptype: Head (m) vs. Vol. Flow Rate (m³/hr) | Pressure (kPa) vs. Vol. Flow Rate (m³/hr) | Pressure (bar) vs. Vol. Flow Rate (m³/hr)
      mask Callback maptype:
      | h      = get_param(gcb,'handle');   % Get block handle
      | blk    = gcb;
      | hblock = get(h);     % Parse out handles structure
      | 
      | if strcmp(hblock.maptype,'Head (m) vs. Vol. Flow Rate (m³/hr)') == 1;
      |     set_param([blk,'/switchcase'],'Value','1');
      |     set_param([blk,'/Pump Vol. FlowRate'],'Table',['PumpProp.',hblock.map,'.q']);
      |     set_param([blk,'/Pump Vol. FlowRate'],'BreakpointsForDimension1',['PumpProp.',hblock.map,'.head']);
      | elseif strcmp(hblock.maptype,'Pressure (kPa) vs. Vol. Flow Rate (m³/hr)') == 1;
      |     set_param([blk,'/switchcase'],'Value','2');
      |     set_param([blk,'/Pump Vol. FlowRate'],'Table',['PumpProp.',hblock.map,'.q']);
      |     set_param([blk,'/Pump Vol. FlowRate'],'BreakpointsForDimension1',['PumpProp.',hblock.map,'.pres']);
      | elseif strcmp(hblock.maptype,'Pressure (bar) vs. Vol. Flow Rate (m³/hr)') == 1;
      |     set_param([blk,'/switchcase'],'Value','3');
      |     set_param([blk,'/Pump Vol. FlowRate'],'Table',['PumpProp.',hblock.map,'.q']);
      |     set_param([blk,'/Pump Vol. FlowRate'],'BreakpointsForDimension1',['PumpProp.',hblock.map,'.pres']);
      | else
      |     error('see pump mask callback for map type');
      | end
      | 
      | clear h blk hblock
      mask TypeOptions map: B737_mech_fuel1 | B737_mech_fuel2 | B737_mech_fuel3 | B737_AC_fuel1 | B737_AC_oil1
      mask Callback map:
      | h      = get_param(gcb,'handle');   % Get block handle
      | blk    = gcb;
      | hblock = get(h);     % Parse out handles structure
      | vals = get_param(blk,'MaskValues');
      | % find all installed pumps in the PumpProp.mat file
      | pumps = fieldnames(PumpProp);
      | indx = strfind(pumps, 'units');
      | indx = find(not(cellfun('isempty', indx)));
      | pumps(indx) = [];      % removing the units entry
      | 
      | for i = 1:size(pumps,1);
      |    if i==1;
      |     pmpstr = pumps{i};
      |    else
      |        pmpstr = strcat(pmpstr,char(124),pumps{i});
      |    end
      | end
      | 
      | % Get the mask parameter values. This is a cell array of strings.
      | styl = get_param(blk,'MaskStyles');
      | 
      | vis = get_param(blk,'MaskVisibilities');
      | str = get_param(blk,'MaskPromptString');
      | 
      | % fill the mask with the parameters
      | set_param(blk,'MaskVisibilities',vis,'MaskPromptString',str,'MaskValues',vals,'MaskStyles',[styl(1);strcat('popup(',pmpstr,')');styl(3:9)]);
      | 
      | clear h blk hblock styl vals vis str pmpstr i indx pumps
      mask Callback AC_pwr:
      | h      = get_param(gcb,'handle');   % Get block handle
      | blk    = gcb;
      | hblock = get(h);     % Parse out handles structure
      | 
      | vis = get_param(blk,'MaskVisibilities');
      | 
      | if strcmp(hblock.AC_pwr,'off') == 1;
      |     % fill the mask with the parameters
      |     set_param(blk,'MaskVisibilities',[vis(1:7);'off';vis(9)])
      |     set_param(blk,'mech_pwr','on');
      |     set_param([blk,'/pwr_switch'],'Value','0.5')
      | elseif strcmp(hblock.AC_pwr,'on') == 1;
      |     % fill the mask with the parameters
      |     set_param(blk,'MaskVisibilities',[vis(1:7);'on';vis(9)])
      |     set_param(blk,'mech_pwr','off');
      |     set_param([blk,'/pwr_switch'],'Value','0')
      | end
      | 
      | clear h blk hblock vis
      mask Callback mech_pwr:
      | h      = get_param(gcb,'handle');   % Get block handle
      | blk    = gcb;
      | hblock = get(h);     % Parse out handles structure
      | 
      | vis = get_param(blk,'MaskVisibilities');
      | 
      | if strcmp(hblock.mech_pwr,'off') == 1;
      |     % fill the mask with the parameters
      |     set_param(blk,'MaskVisibilities',[vis(1:7);'on';vis(9)])
      |     set_param(blk,'AC_pwr','on');
      |     set_param([blk,'/pwr_switch'],'Value','0')
      | elseif strcmp(hblock.mech_pwr,'on') == 1;
      |     % fill the mask with the parameters
      |     set_param(blk,'MaskVisibilities',[vis(1:7);'off';vis(9)])
      |     set_param(blk,'AC_pwr','off');
      |     set_param([blk,'/pwr_switch'],'Value','0.5')
      | end
      | clear h blk hblock vis
      mask Display:
      | image(imread('centpump.jpg'));
      | 
      | port_label('input',1,'{\bf Flow In}','TexMode','on')
      | port_label('input',2,'{\bf w (rpm)}','TexMode','on')
      | port_label('input',3,'{\bf P_o_u_t (kPa)}','TexMode','on')
      | 
      | port_label('output',1,'{\bf Flow Out}','TexMode','on')
      | port_label('output',2,'{\bf Pump Power}','TexMode','on')
      | 
      | h      = get_param(gcb,'handle');   % Get block handle
      | hblock = get(h);     % Parse out handles structure
      | 
      | if heat_out == 0
      |     port_label('output',3,'{\bf Pump Heat [kW]}','TexMode','on')
      | end
  Right Wing Fuel Pump  #6 : Subsystem  AncestorBlock=PowerFlowLib/Energy & Power Systems/Thermal/Fuel/Fuel Pump  mask(Pump){maptype=Pressure (kPa) vs. Vol. Flow Rate (m³/hr), map=B737_AC_fuel1, map_load=off, SG=0.82, pump_eff=.75, heat_out=off, AC_pwr=on, pf=1, mech_pwr=off}
      mask prompts: maptype "Map Type"; map "Select Map"; map_load "Load new map?"; SG "Specific Gravity of Flow"; pump_eff "Pump Overall Efficiency"; heat_out "Add heat to flow?"; AC_pwr "AC Powered?"; pf "Power Factor"; mech_pwr "Mechanically Driven?"
      mask help:
      | Input 1: Input Flow Bus
      | Input 2: Shaft RPM (rpm)
      | Input 3: Upstream Pressure (kPa)
      |
      | Output 1: Output Flow Bus
      | Output 2: Pump Power Bus (mech or elec)
      | Optional: Pump Heat Generated (kW)
      mask init: same as ECS_FOS/ECS/Fuel Tanks/Pumps/Right Wing Fuel Pump  #1
      settings: OpenFcn=|
      | if exist('PumpProp') == 0
      |   load('PumpProp.mat')
      | end
      | open_system(gcb,'mask')
      mask TypeOptions maptype: Head (m) vs. Vol. Flow Rate (m³/hr) | Pressure (kPa) vs. Vol. Flow Rate (m³/hr) | Pressure (bar) vs. Vol. Flow Rate (m³/hr)
      mask Callback maptype:
      | h      = get_param(gcb,'handle');   % Get block handle
      | blk    = gcb;
      | hblock = get(h);     % Parse out handles structure
      | 
      | if strcmp(hblock.maptype,'Head (m) vs. Vol. Flow Rate (m³/hr)') == 1;
      |     set_param([blk,'/switchcase'],'Value','1');
      |     set_param([blk,'/Pump Vol. FlowRate'],'Table',['PumpProp.',hblock.map,'.q']);
      |     set_param([blk,'/Pump Vol. FlowRate'],'BreakpointsForDimension1',['PumpProp.',hblock.map,'.head']);
      | elseif strcmp(hblock.maptype,'Pressure (kPa) vs. Vol. Flow Rate (m³/hr)') == 1;
      |     set_param([blk,'/switchcase'],'Value','2');
      |     set_param([blk,'/Pump Vol. FlowRate'],'Table',['PumpProp.',hblock.map,'.q']);
      |     set_param([blk,'/Pump Vol. FlowRate'],'BreakpointsForDimension1',['PumpProp.',hblock.map,'.pres']);
      | elseif strcmp(hblock.maptype,'Pressure (bar) vs. Vol. Flow Rate (m³/hr)') == 1;
      |     set_param([blk,'/switchcase'],'Value','3');
      |     set_param([blk,'/Pump Vol. FlowRate'],'Table',['PumpProp.',hblock.map,'.q']);
      |     set_param([blk,'/Pump Vol. FlowRate'],'BreakpointsForDimension1',['PumpProp.',hblock.map,'.pres']);
      | else
      |     error('see pump mask callback for map type');
      | end
      | 
      | clear h blk hblock
      mask TypeOptions map: B737_mech_fuel1 | B737_mech_fuel2 | B737_mech_fuel3 | B737_AC_fuel1 | B737_AC_oil1
      mask Callback map:
      | h      = get_param(gcb,'handle');   % Get block handle
      | blk    = gcb;
      | hblock = get(h);     % Parse out handles structure
      | vals = get_param(blk,'MaskValues');
      | % find all installed pumps in the PumpProp.mat file
      | pumps = fieldnames(PumpProp);
      | indx = strfind(pumps, 'units');
      | indx = find(not(cellfun('isempty', indx)));
      | pumps(indx) = [];      % removing the units entry
      | 
      | for i = 1:size(pumps,1);
      |    if i==1;
      |     pmpstr = pumps{i};
      |    else
      |        pmpstr = strcat(pmpstr,char(124),pumps{i});
      |    end
      | end
      | 
      | % Get the mask parameter values. This is a cell array of strings.
      | styl = get_param(blk,'MaskStyles');
      | 
      | vis = get_param(blk,'MaskVisibilities');
      | str = get_param(blk,'MaskPromptString');
      | 
      | % fill the mask with the parameters
      | set_param(blk,'MaskVisibilities',vis,'MaskPromptString',str,'MaskValues',vals,'MaskStyles',[styl(1);strcat('popup(',pmpstr,')');styl(3:9)]);
      | 
      | clear h blk hblock styl vals vis str pmpstr i indx pumps
      mask Callback AC_pwr:
      | h      = get_param(gcb,'handle');   % Get block handle
      | blk    = gcb;
      | hblock = get(h);     % Parse out handles structure
      | 
      | vis = get_param(blk,'MaskVisibilities');
      | 
      | if strcmp(hblock.AC_pwr,'off') == 1;
      |     % fill the mask with the parameters
      |     set_param(blk,'MaskVisibilities',[vis(1:7);'off';vis(9)])
      |     set_param(blk,'mech_pwr','on');
      |     set_param([blk,'/pwr_switch'],'Value','0.5')
      | elseif strcmp(hblock.AC_pwr,'on') == 1;
      |     % fill the mask with the parameters
      |     set_param(blk,'MaskVisibilities',[vis(1:7);'on';vis(9)])
      |     set_param(blk,'mech_pwr','off');
      |     set_param([blk,'/pwr_switch'],'Value','0')
      | end
      | 
      | clear h blk hblock vis
      mask Callback mech_pwr:
      | h      = get_param(gcb,'handle');   % Get block handle
      | blk    = gcb;
      | hblock = get(h);     % Parse out handles structure
      | 
      | vis = get_param(blk,'MaskVisibilities');
      | 
      | if strcmp(hblock.mech_pwr,'off') == 1;
      |     % fill the mask with the parameters
      |     set_param(blk,'MaskVisibilities',[vis(1:7);'on';vis(9)])
      |     set_param(blk,'AC_pwr','on');
      |     set_param([blk,'/pwr_switch'],'Value','0')
      | elseif strcmp(hblock.mech_pwr,'on') == 1;
      |     % fill the mask with the parameters
      |     set_param(blk,'MaskVisibilities',[vis(1:7);'off';vis(9)])
      |     set_param(blk,'AC_pwr','off');
      |     set_param([blk,'/pwr_switch'],'Value','0.5')
      | end
      | clear h blk hblock vis
      mask Display:
      | image(imread('centpump.jpg'));
      | 
      | port_label('input',1,'{\bf Flow In}','TexMode','on')
      | port_label('input',2,'{\bf w (rpm)}','TexMode','on')
      | port_label('input',3,'{\bf P_o_u_t (kPa)}','TexMode','on')
      | 
      | port_label('output',1,'{\bf Flow Out}','TexMode','on')
      | port_label('output',2,'{\bf Pump Power}','TexMode','on')
      | 
      | h      = get_param(gcb,'handle');   % Get block handle
      | hblock = get(h);     % Parse out handles structure
      | 
      | if heat_out == 0
      |     port_label('output',3,'{\bf Pump Heat [kW]}','TexMode','on')
      | end
  Right Wing Fuel Tank : Subsystem  AncestorBlock=PowerFlowLib/Energy & Power Systems/Thermal/Fuel/Fuel Tank  mask(Fuel Tank){fileslct=off, filename=fueltank_area.m, filedir=C:\Users\mwillms4\Documents\My Box Files\Graduate\Research\PowerFlow Development\PowerFlow Fall 2013\SupportFunctions\fueltank_area.m, tank_loc=Right Wing Tank, areaprompt2=off, max_vol=3.2, m_init=2500, fld_Tint=0, ull_Tint=30, Pover=100, HTC_fg=14.2, wallHXF=off, wetHTC=14.2, dryHTC=14.2, Qinternal=0}
      mask prompts: fileslct "Browse for area .m file?"; filename "Fuel Tank Area .m File"; filedir "Area .m File Directory"; tank_loc "Select Tank"; areaprompt2 "Edit Fuel Tank Area Manually?"; max_vol "Maximum Tank Volume [m³]"; m_init "Initial Fluid Mass [kg]"; fld_Tint "Initial Fluid Temperature [°C]"; ull_Tint "Initial Ullage Temperature [°C]"; Pover "Tank Pressurization [kPa]"; HTC_fg "Fuel to Ullage HTC [W/m² K]"; wallHXF "Enable Wall Heat Transfer"; wetHTC "Wall to Fluid HTC [W/m² K]"; dryHTC "Wall to Ullage HTC [W/m² K]"; Qinternal "Internal Heat Load [W]"
      mask help:
      | Input 1: Input Flow Bus
      | Input 2: Flow Rate Out [kg/s]
      | Input 3: Ambient Pressure [kPa]
      | Input 4: Heat Load [W]
      | Input 5: Initial Wall Temps. Vector [K]
      |
      | Output 1: Output Flow Bus
      | Output 2: Tank mass [kg]
      | Output 3: Ullage Temp. [K]
      mask init: same as ECS_FOS/ECS/Fuel Tanks/Pumps/Center Fuel Tank
      mask Callback fileslct:
      | h      = get_param(gcb,'handle');   % Get block handle
      | blk    = gcb;
      | hblock = get(h);     % Parse out handles structure
      | 
      | if strcmp(hblock.fileslct,'on') == 1;
      |     set_param(gcb,'areaprompt2','off');     % turn off manual switch
      |     RR_SetPerfSlct(2,0);                    % call uiopen script
      | end
      | 
      | clear h blk hblock
      mask TypeOptions tank_loc: Left Wing Tank | Center Tank | Right Wing Tank
      mask Callback areaprompt2:
      | h      = get_param(gcb,'handle');   % Get block handle
      | blk    = gcb;
      | hblock = get(h);     % Parse out handles structure
      | 
      | if strcmp(hblock.areaprompt2,'on') == 1;
      |     set_param(gcb,'fileslct','off');
      |     open_system([blk, '/Wall Heat Transfer/volume_%']);
      | end
      mask Callback wallHXF:
      | h      = get_param(gcb,'handle');   % Get block handle
      | blk    = gcb;
      | hblock = get(h);     % Parse out handles structure
      | 
      | if strcmp(hblock.wallHXF,'on') == 1;
      |     set_param([blk,'/enable_wall_HXF'],'Value','1');
      | else
      |     set_param([blk,'/enable_wall_HXF'],'Value','0');
      | end
      | 
      | clear h blk hblock
      mask Display:
      | image(imread('fueltank.jpg'))
      | 
      | port_label('input',1,'{\bf Flow In}','TexMode','on')
      | port_label('input',2,'{\bf Flow Rate Out}','TexMode','on')
      | port_label('input',3,'{\bf P_a_m_b [kPa]}','TexMode','on')
      | port_label('input',4,'{\bf Heat Load [kW]}','TexMode','on')
      | port_label('input',5,'{\bf Wall Temp. [K]}','TexMode','on')
      | 
      | port_label('output',1,'{\bf Flow Out }','TexMode','on')
      | port_label('output',2,'{\bf Fluid Mass [kg]}','TexMode','on')
      | port_label('output',3,'{\bf Ullage Temp. [K]}','TexMode','on')
  Scope{,1..5} (6 alike) : Scope
      Scope settings: SaveName=ScopeData21
      Scope1 settings: YMin=2498.9  YMax=2498.9  SaveName=ScopeData23
      Scope2 settings: SaveName=ScopeData25
      Scope3 settings: SaveName=ScopeData27
      Scope4 settings: SaveName=ScopeData28
      Scope5 settings: SaveName=ScopeData29
  Terminator{,1..5} (6 alike) : Terminator
  Fuel Left Wing : Outport
  Fuel Right  Wing : Outport  Port=2
  wires:
  Right Wing Fuel Pump  #6/3(Heat (kW)) -> Add6/2
  Right Wing Fuel Pump  #5/3(Heat (kW)) -> Add6/1
  Right Wing Fuel Pump  #4/3(Heat (kW)) -> Add4/2
  Right Wing Fuel Pump  #3/3(Heat (kW)) -> Add4/1
  Right Wing Fuel Pump  #2/3(Heat (kW)) -> Add3/2
  Right Wing Fuel Pump  #1/3(Heat (kW)) -> Add3/1
  Bus Selector10/2 -> ElectricalSink6/2  "<react_pwr_VAr>"
  Bus Selector10/1 -> ElectricalSink6/1  "<real_pwr_W>"
  Bus Selector9/2 -> ElectricalSink5/2  "<react_pwr_VAr>"
  Bus Selector9/1 -> ElectricalSink5/1  "<real_pwr_W>"
  Bus Selector7/2 -> ElectricalSink4/2  "<react_pwr_VAr>"
  Bus Selector7/1 -> ElectricalSink4/1  "<real_pwr_W>"
  Bus Selector6/2 -> ElectricalSink3/2  "<react_pwr_VAr>"
  Bus Selector6/1 -> ElectricalSink3/1  "<real_pwr_W>"
  Bus Selector4/2 -> ElectricalSink2/2  "<react_pwr_VAr>"
  Bus Selector4/1 -> ElectricalSink2/1  "<real_pwr_W>"
  Bus Selector2/2 -> ElectricalSink1/2  "<react_pwr_VAr>"
  Right Wing Fuel Pump  #1/2(Pump Power) -> Bus Selector2/1
  Add3/1 -> [heat_tank_rght]
  Add4/1 -> [heat_tank_cen]
  Bus Selector2/1 -> ElectricalSink1/1  "<real_pwr_W>"
  Bus Selector15/1 -> [Fuel_RWing]  "<FuelFlowNeed_kgps>"
  Fuel Demand  Right Wing/1 -> Bus Selector15/1
  Bus Selector/1 -> [Fuel_LWing]  "<FuelFlowNeed_kgps>"
  Pump Split3/1(Flow Out) -> Right Wing Fuel Pump  #6/1(Flow_in), Right Wing Fuel Pump  #5/1(Flow_in)
  Fuel Control Left Wing/1(Fuel2Engine) -> Fuel Left Wing/1
  "Fuel Control Right Wing "/1(Fuel2Engine) -> Fuel Right  Wing/1
  "Fuel Control Right Wing "/2(Fuel2Tank) -> [rw_fuel_rtrn]
  Fuel Control Left Wing/2(Fuel2Tank) -> [lw_fuel_rtrn]
  [Fuel_LWing] -> Fuel Control Left Wing/1(FuelNeed)
  [Fuel_RWing] -> "Fuel Control Right Wing "/1(FuelNeed)
  Fuel Demand  Left Wing/1 -> Bus Selector/1
  Ground2/1 -> Left Wing Fuel Tank/5(Wall_temps)
  Ground1/1 -> Center Fuel Tank/5(Wall_temps)
  Ground/1 -> Right Wing Fuel Tank/5(Wall_temps)
  Left Wing Fuel Tank/3(ullage_T) -> Terminator5/1
  Left Wing Fuel Tank/2(fluid_mass) -> Terminator4/1
  Center Fuel Tank/3(ullage_T) -> Terminator3/1
  Center Fuel Tank/2(fluid_mass) -> Scope2/1, Terminator2/1
  Right Wing Fuel Tank/3(ullage_T) -> Terminator1/1
  Right Wing Fuel Tank/2(fluid_mass) -> Scope1/1, Terminator/1
  [Fuel_RWing] -> Scope/1, Flow Junction/1
  [Fuel_LWing] -> Flow Junction1/1
  [pres_rght] -> Right Wing Fuel Pump  #1/3(P_out)
  [pres_rght] -> Right Wing Fuel Pump  #2/3(P_out)
  [pres_rght] -> Right Wing Fuel Pump  #3/3(P_out)
  [pres_lft] -> Right Wing Fuel Pump  #4/3(P_out)
  [pres_lft] -> Right Wing Fuel Pump  #6/3(P_out)
  [pres_lft] -> Right Wing Fuel Pump  #5/3(P_out)
  Bus Selector14/1 -> [pres_lft]  "<pres_kPa>"
  [lw_rpm] -> Right Wing Fuel Pump  #6/2(w_rpm)
  [lw_rpm] -> Right Wing Fuel Pump  #5/2(w_rpm)
  [cen_rpm] -> Right Wing Fuel Pump  #4/2(w_rpm)
  [cen_rpm] -> Right Wing Fuel Pump  #3/2(w_rpm)
  [rw_rpm] -> Right Wing Fuel Pump  #2/2(w_rpm)
  Bus Selector13/1 -> [pres_rght]  "<pres_kPa>"
  [heat_tank_rght] -> Right Wing Fuel Tank/4(Heat load)
  [heat_tank_cen] -> Center Fuel Tank/4(Heat load)
  [heat_tank_lft] -> Left Wing Fuel Tank/4(Heat load)
  Add6/1 -> [heat_tank_lft]
  [Pres_Amb_kPa] -> Left Wing Fuel Tank/3(Pamb)
  [Pres_Amb_kPa] -> Center Fuel Tank/3(Pamb)
  [Pres_Amb_kPa] -> Right Wing Fuel Tank/3(Pamb)
  Add2/1 -> [mdot_tank_cen]  "mdot_kgps"
  Bus Selector11/1 -> Add2/1  "<mdot_kgps>"
  Bus Selector12/1 -> Add2/2  "<mdot_kgps>"
  Add1/1 -> [mdot_tank_lft]  "mdot_kgps"
  Bus Selector1/1 -> Add1/1  "<mdot_kgps>"
  Bus Selector3/1 -> Add1/2  "<mdot_kgps>"
  Add5/1 -> [mdot_tank_rght]  "mdot_kgps"
  Bus Selector5/1 -> Add5/1  "<mdot_kgps>"
  Left Wing Fuel Tank/1(Flow_Out) -> Pump Split3/1(Flow In)
  Pump Split2/1(Flow Out) -> Right Wing Fuel Pump  #4/1(Flow_in), Right Wing Fuel Pump  #3/1(Flow_in)
  [mdot_tank_lft] -> Left Wing Fuel Tank/2(Flow Out)
  [mdot_tank_cen] -> Center Fuel Tank/2(Flow Out)
  [mdot_tank_rght] -> Right Wing Fuel Tank/2(Flow Out)
  Bus Selector8/1 -> Add5/2  "<mdot_kgps>"
  Pump Split1/1(Flow Out) -> Right Wing Fuel Pump  #2/1(Flow_in), Right Wing Fuel Pump  #1/1(Flow_in)
  Right Wing Fuel Tank/1(Flow_Out) -> Pump Split1/1(Flow In)
  [rw_rpm] -> Right Wing Fuel Pump  #1/2(w_rpm)
  Right Wing Fuel Pump  #1/1(Flow_Out) -> Scope3/1, Flow Junction/2, Bus Selector5/1
  Right Wing Fuel Pump  #2/2(Pump Power) -> Bus Selector4/1
  [rw_fuel_rtrn] -> Right Wing Fuel Tank/1(Flow)
  Right Wing Fuel Pump  #2/1(Flow_Out) -> Scope4/1, Flow Junction/3, Bus Selector8/1
  Center Fuel Tank/1(Flow_Out) -> Pump Split2/1(Flow In)
  Flow Junction/1 -> "Fuel Control Right Wing "/2(FuelFromPump), Bus Selector13/1  "to right wing engine"
  Right Wing Fuel Pump  #3/2(Pump Power) -> Bus Selector6/1
  Right Wing Fuel Pump  #3/1(Flow_Out) -> Scope5/1, Flow Junction/4, Bus Selector11/1
  Flow Junction1/1 -> Fuel Control Left Wing/2(FuelFromPump), Bus Selector14/1  "to left wing engine"
  Right Wing Fuel Pump  #4/2(Pump Power) -> Bus Selector7/1
  FlowGenerator1/1(FlowOut) -> Center Fuel Tank/1(Flow)
  Right Wing Fuel Pump  #4/1(Flow_Out) -> Flow Junction1/2, Bus Selector12/1
  Right Wing Fuel Pump  #5/2(Pump Power) -> Bus Selector9/1
  Right Wing Fuel Pump  #5/1(Flow_Out) -> Flow Junction1/3, Bus Selector1/1
  Right Wing Fuel Pump  #6/2(Pump Power) -> Bus Selector10/1
  [lw_fuel_rtrn] -> Left Wing Fuel Tank/1(Flow)
  Right Wing Fuel Pump  #6/1(Flow_Out) -> Flow Junction1/4, Bus Selector3/1
  Fuel Switch On/Off/3(Center RPM) -> [cen_rpm]
  Fuel Switch On/Off/2(Left Wing RPM) -> [lw_rpm]
  Fuel Switch On/Off/1(Right Wing RPM) -> [rw_rpm]
  Fuel Switch2/1 -> Fuel Switch On/Off/3(Left Wing Tank)
  Fuel Switch1/1 -> Fuel Switch On/Off/2(Center Tank)
  Fuel Switch/1 -> Fuel Switch On/Off/1(Right Wing Tank)
  Pamb/1 -> [Pres_Amb_kPa]
